simulink model "slink"  (Simulink 10.1)
settings: Solver=ode45  StartTime=0.0  StopTime=10  RelTol=1e-3  EnableMultiTasking=on
values from neighbouring files (symbols this model uses):
  Ao = [1.38 -0.2077 6.715 -5.676 ... (first row only)    [sslabsc.m]
  Bo = [0 0; 5.679 0; 1.136 -3.146; 1.136 0]    [sslabsc.m]
  Co = [1 0 0 0; 0 1 0 0; 0 0 1 -1]    [sslabsc.m]
  Do = zeros(3,2)    [sslabsc.m]
  K = place(A,B,eig_cl)    [main.m]    (also in sslabsc.m = zeros(2,4))
settings Model: Creator=bjones  LastModifiedBy=ACER  ExtModeTrigMode=oneshot  ExtModeArmWhenConnect=off
settings DataIOCC: SignalLoggingSaveFormat=ModelDataLogs
settings OptimizationCC: BlockReduction=off  BooleanDataType=off  ExpressionDepthLimit=2147483647  InitFltsAndDblsToZero=on
settings DebuggingCC: SaveWithParameterizedLinksMsg=none  SignalResolutionControl=TryResolveAllWithWarning  MultiTaskDSMMsg=warning  MultiTaskCondExecSysMsg=none  FcnCallInpInsideContextMsg=warning  StateNameClashWarn=warning
settings HardwareCC: TargetUnknown=on
settings GRTTargetCC: TargetFcnLib=ansi_tfl_tmw.mat  ModelReferenceCompliant=off  ParMdlRefBuildCompliant=off  CompOptLevelCompliant=off  MatFileLogging=off

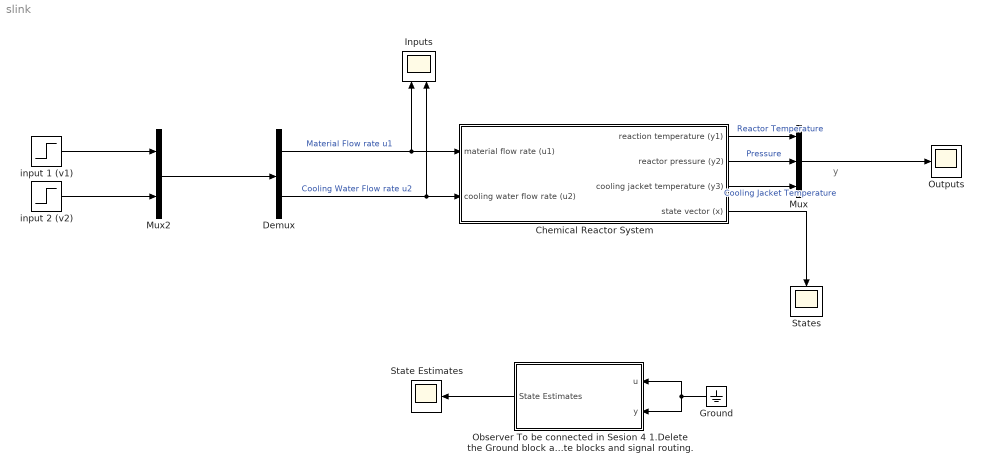
== system slink ==
  note: y
  Chemical Reactor System : Subsystem  mask(System Block){}
      mask help: Chemical reactor system used for the ACS6129 laboratory. Please ask a demonstrator or press help if you are interested in the underlying workings of the system.
      mask Help:
      | This is the chemical reactor system block for use in the ACS6129 laboratory. This block implements a continuous time state space model of the system, using a set of pre-defined system matrices found in the sslabsc.m file.
      | 
      | This block should not be edited, and for further information about the block please ask a demonstrator.
  Demux : Demux  Outputs=2
  Ground : Ground
  Inputs : Scope  NumInputPorts=2
  Mux : Mux  Inputs=3
  Mux2 : Mux  Inputs=2
  "Observer To be connected in Sesion 4 1.Delete the Ground block and connect the inputs of the observer to the appropriate signal channels 2. Double click on the observer block to open it. 3. Complete the implementation of the observer  by using appropriate blocks and signal routing. " : Subsystem
  Outputs : Scope
  State Estimates : Scope
  States : Scope
  input 1 (v1) : Step  SampleTime=0
  input 2 (v2) : Step  SampleTime=0
  wires:
  input 1 (v1)/1 -> Mux2/1
  input 2 (v2)/1 -> Mux2/2
  Chemical Reactor System/4(state vector (x)) -> States/1
  Chemical Reactor System/1(reaction temperature (y1)) -> Mux/1  "Reactor Temperature"
  Chemical Reactor System/2(reactor pressure (y2)) -> Mux/2  "Pressure"
  Chemical Reactor System/3(cooling jacket temperature (y3)) -> Mux/3  "Cooling Jacket Temperature"
  Mux/1 -> Outputs/1
  Demux/1 -> Chemical Reactor System/1(material flow rate (u1)), Inputs/1  "Material Flow rate u1"
  Demux/2 -> Chemical Reactor System/2(cooling water flow rate (u2)), Inputs/2  "Cooling Water Flow rate u2"
  "Observer To be connected in Sesion 4 1.Delete the Ground block and connect the inputs of the observer to the appropriate signal channels 2. Double click on the observer block to open it. 3. Complete the implementation of the observer  by using appropriate blocks and signal routing. "/1(State Estimates) -> State Estimates/1
  Ground/1 -> "Observer To be connected in Sesion 4 1.Delete the Ground block and connect the inputs of the observer to the appropriate signal channels 2. Double click on the observer block to open it. 3. Complete the implementation of the observer  by using appropriate blocks and signal routing. "/1(u), "Observer To be connected in Sesion 4 1.Delete the Ground block and connect the inputs of the observer to the appropriate signal channels 2. Double click on the observer block to open it. 3. Complete the implementation of the observer  by using appropriate blocks and signal routing. "/2(y)
  Mux2/1 -> Demux/1

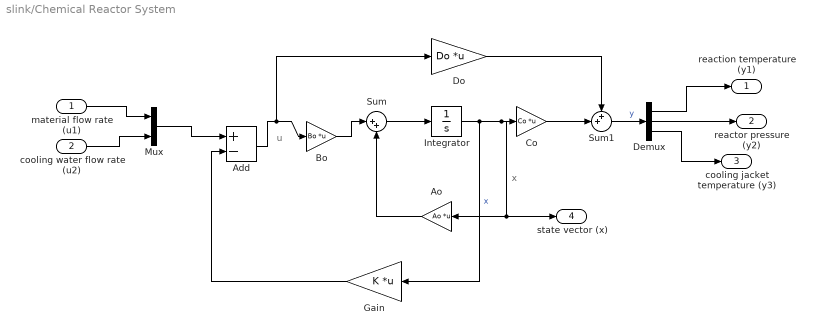
== system slink/Chemical Reactor System ==
  note: u
  note: x
  material flow rate (u1) : Inport
  cooling water flow rate (u2) : Inport  Port=2
  Add : Sum  Inputs=+-
  Ao : Gain  Gain=Ao  Multiplication=Matrix(K*u)  SaturateOnIntegerOverflow=on  OutDataTypeStr=Inherit: Same as input  ParamDataTypeStr=Inherit: Same as input
  Bo : Gain  Gain=Bo  Multiplication=Matrix(K*u)  SaturateOnIntegerOverflow=on  OutDataTypeStr=Inherit: Same as input  ParamDataTypeStr=Inherit: Same as input
  Co : Gain  Gain=Co  Multiplication=Matrix(K*u)  SaturateOnIntegerOverflow=on  OutDataTypeStr=Inherit: Same as input  ParamDataTypeStr=Inherit: Same as input
  Demux : Demux  Outputs=3
  Do : Gain  Gain=Do  Multiplication=Matrix(K*u)  SaturateOnIntegerOverflow=on  OutDataTypeStr=Inherit: Same as input  ParamDataTypeStr=Inherit: Same as input
  Gain : Gain  Gain=K  Multiplication=Matrix(K*u)
  Integrator : Integrator
  Mux : Mux  Inputs=2
  Sum : Sum  Inputs=|++  InputSameDT=on  SaturateOnIntegerOverflow=on  OutDataTypeStr=Inherit: Same as first input
  Sum1 : Sum  Inputs=++|  InputSameDT=on  SaturateOnIntegerOverflow=on  OutDataTypeStr=Inherit: Same as first input
  reaction temperature (y1) : Outport
  reactor pressure (y2) : Outport  Port=2
  cooling jacket temperature (y3) : Outport  Port=3
  state vector (x) : Outport  Port=4
  wires:
  Integrator/1 -> Gain/1, Co/1, Ao/1, state vector (x)/1  "x"
  Sum/1 -> Integrator/1
  Bo/1 -> Sum/1
  Ao/1 -> Sum/2
  Do/1 -> Sum1/1
  Co/1 -> Sum1/2
  material flow rate (u1)/1 -> Mux/1
  cooling water flow rate (u2)/1 -> Mux/2
  Sum1/1 -> Demux/1  "y"
  Demux/1 -> reaction temperature (y1)/1
  Demux/2 -> reactor pressure (y2)/1
  Demux/3 -> cooling jacket temperature (y3)/1
  Add/1 -> Do/1, Bo/1
  Mux/1 -> Add/1
  Gain/1 -> Add/2

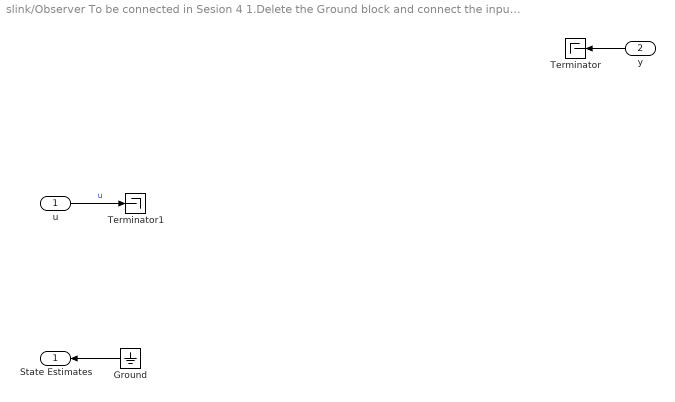
== system slink/Observer To be connected in Sesion 4 1.Delete the Ground block and connect the inputs of the observer to the appropriate signal channels 2. Double click on the observer block to open it. 3. Complete the implementation of the observer  by using appropriate blocks and signal routing.  ==
  u : Inport
  y : Inport  Port=2
  Ground : Ground
  Terminator : Terminator
  Terminator1 : Terminator
  State Estimates : Outport
  wires:
  y/1 -> Terminator/1
  u/1 -> Terminator1/1  "u"
  Ground/1 -> State Estimates/1
